simulink model "L7_Project_218"  (R2021b)
settings: Solver=VariableStepAuto  StartTime=0.0  StopTime=0.2  RelTol=1e-3
values from neighbouring files (symbols this model uses):
  Ts = T_pwm    (= 0.001)    [RLagent.m]
  Ts_agent = Ts    (= 0.001)    [RLagent.m]
  Ts_simulink = T_pwm/2    (= 0.0005)    [RLagent.m]
  Ts_speed = 10*Ts    (= 0.01)    [RLagent.m]
undefined symbols (not defined in the file or in its folder): DiscIntNeverNeededParam
libraries: spsIGBTLib x6, spsSeriesRLCBranchLib x6, mcbcontrolslib x3, simulink x2, spsDCVoltageSourceLib x1, spsPermanentMagnetSynchronousMachineLib x1, eePmsmTorqueEstimator x1, rllib x1, spsThreePhaseVIMeasurementLib x1, spspowerguiLib x1
settings Model: Creator=HP  LastModifiedBy=HP
settings DebuggingCC: ParameterPrecisionLossMsg=none

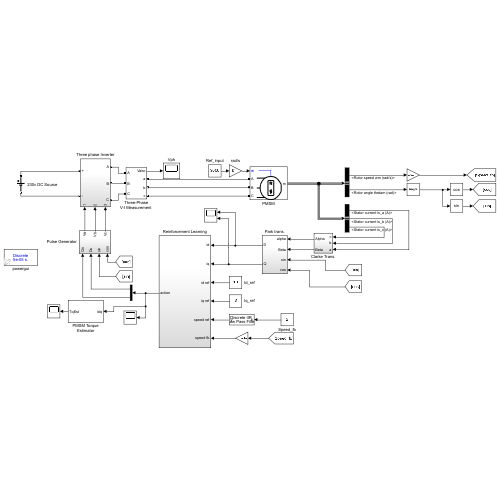
[thumbnail: Simulink's stored preview of the top-level diagram]
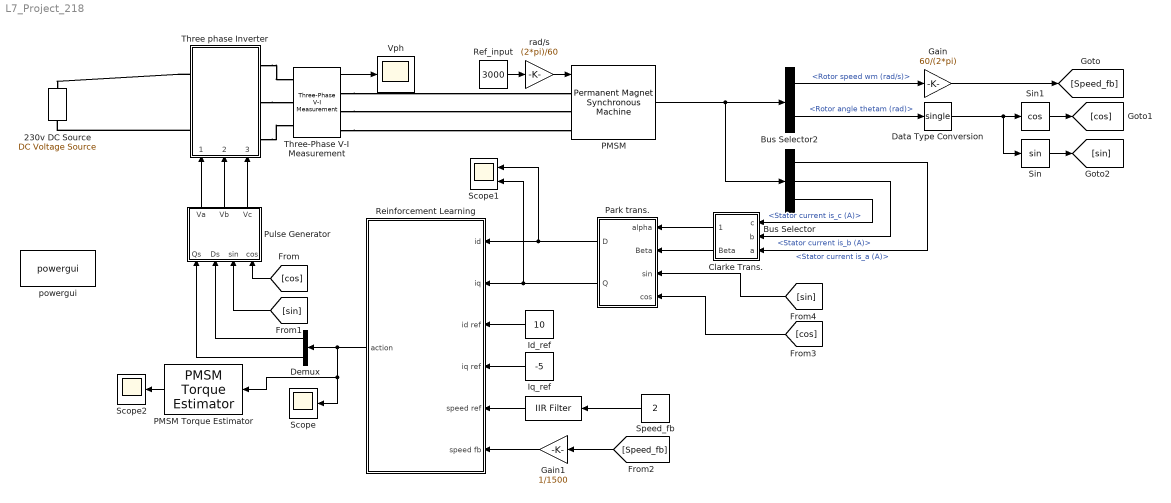
== system L7_Project_218 ==
  "   " : mcbcontrolslib/IIR Filter  VariantControl=Low Pass Filter  VariantSelect=Low-pass  Filter_constant=0.01*(Ts_speed/Ts)  advancedSettings=off  Ts=50e-6  cutOff_freq=353.6777
      settings: SourceProductBaseCode=MT
  230v DC Source : spsDCVoltageSourceLib/DC Voltage Source  Amplitude=230  Measurements=None
  Bus Selector : BusSelector  OutputSignals=Stator current is_a (A),Stator current is_b (A),Stator current is_c (A)
  Bus Selector2 : BusSelector  OutputSignals=Rotor speed wm (rad/s),Rotor angle thetam (rad)
  Clarke Trans. : Subsystem
  Data Type Conversion : DataTypeConversion  OutDataTypeStr=single
  Demux : Demux  Outputs=2
  Gain : Gain  Gain=60/(2*pi)  OutDataTypeStr=double
  Gain1 : Gain  Gain=1/1500
  Id_ref : Constant  Value=10  OutDataTypeStr=double  SampleTime=Ts_speed
  Iq_ref : Constant  Value=-5  OutDataTypeStr=double  SampleTime=Ts_speed
  PMSM : spsPermanentMagnetSynchronousMachineLib/Permanent Magnet Synchronous Machine  NbPhases=3  FluxDistribution=Sinusoidal  RotorType=Salient-pole  MechanicalLoad=Speed w  PresetModel=No  ShowDetailedParameters=on  MeasurementBus=off  Resistance=18.7  Inductance=8.5e-3  dqInductances=[0.02547 0.02816]  La=0.000395  MachineConstant=Flux linkage established by magnets (V.s)  Flux=0.1716  VoltageCst=62.2496  TorqueCst=0.5148  Flat=120  Mechanical=[2.26e-05 1.349e-05 2 0]  PolePairs=2  InitialConditions=[0,0, 0,0]  InitialConditions5ph=[0 0 0 0 0 0]  RefAngle=Aligned with phase A axis (original Park)  IterativeDiscreteModel=Trapezoidal non iterative  TsBlock=-1  TsPowergui=0
  PMSM Torque Estimator : eePmsmTorqueEstimator/PMSM Torque Estimator  ParamType=Constant parameters  p=8  idVect=[-200, 200]  iqVect=[-200, 200]  LdMatrix=0.0002 * ones(2, 2)  LqMatrix=0.0002 * ones(2, 2)  psimMatrix=0.04 * ones(2, 2)  Ld=0.0002  Lq=0.0002  psim=0.04  Ts=-1
      settings: SourceProductBaseCode=PS
  Park trans. : Subsystem
  Pulse Generator : Subsystem
  Ref_input : Constant  Value=3000  SampleTime=Ts_simulink
  Reinforcement Learning : Subsystem
  Scope : Scope
  Scope1 : Scope  NumInputPorts=2
  Scope2 : Scope
  Sin : Trigonometry  NumberOfDataPoints=double
  Sin1 : Trigonometry  Operator=cos
  Speed_fb : Constant  Value=2  SampleTime=Ts_speed
  Three phase Inverter : Subsystem
      settings: PortSchema="{\"entries\":[{\"content\":{\"sides\":[{\"content\":{\"connectorIds\":[\"LConn1\",\"LConn2\"]},\"type\":\"ConnectorPlacement.EquallySpacedRectSide\",\"uuid\":\"7b196236-775e-42c1-83d0-0d6d250710e6\"},{\"content\":{\"connectorIds\":[\"RConn1\",\"RConn2\",\"RConn3\"],\"side\":\"RIGHT\"},\"type\":\"ConnectorPlacement.EquallySpacedRectSide\",\"uuid\":\"b457e177-0c4c-43e7-9cb7-fdd2074136b6\"},{\"content\":{\"connectorIds\":[],\"side\":\"TOP\"},\"type\":\"ConnectorPlacement.EquallySpacedRectSide\",\"uuid\":\"18a8f709-510a-4ef1-9b8b-174ec6aa79c3\"},{\"content\":{\"connectorIds\":[\"In1\",\"In2\",\"In3\"],\"side\":\"BOTTOM\"},\"type\":\"ConnectorPlacement.EquallySpacedRectSide\",\"uuid\":\"6b6fe34a-9a26-41fc-be3f-ad32a70b0e9c\"}]},\"type\":\"ConnectorPlacement.EquallySpacedConnector\",\"uuid\":\"c4aeab25-f1ae-4405-83d3-42d09976eee9\"}],\"packageUris\":[\"http://schema.mathworks.com/mf0/Connector/R2020b\"],\"version\":\"1.0\"}"
  "Three-Phase V-I Measurement " : spsThreePhaseVIMeasurementLib/Three-Phase V-I Measurement  VoltageMeasurement=phase-to-phase  SetLabelV=off  LabelV=Vabc  Vpu=off  VpuLL=off  CurrentMeasurement=no  SetLabelI=off  LabelI=Iabc  Ipu=off  Pbase=100e6  Vbase=500e3  OutputType=Complex  PhasorSimulation=off  PSBequivalent=0
  Vph : Scope
  powergui : spspowerguiLib/powergui  Priority=1  SimulationMode=Discrete  SampleTime=50e-6  frequency=60  Iterations=50  frequencyindice=0  Pbase=100e6  ErrMax=1e-4  UnitsV=kV  UnitsW=MW  buscounter=0  FunctionMessages=off  echomessages=off  EnableUseOfTLC=off  CurrentSourceSwitches=off  DisableSnubberDevices=off  DisableRonSwitches=off  DisableVfSwitches=off  DisplayEquations=off  AutomaticDiscreteSolvers=off  SolverType=Tustin/Backward Euler (TBE)  Interpol=off  ExternalGateDelay=off  methode=off  Ts=100  x0status=blocks  SPID=on  SwTol=0  HookPort=off  NonlinearTolerance=1e-4  nMaxIteration=100  ContinueOnMaxIteration=off  RestoreLinks=warning  ResistiveCurrentMeasurement=off  Frange=[0:2:500]  Ylog=off  Xlog=on  ShowGrid=off  save=off  variable=ZData  structure=0  ZoomFFT=off  StartTime=0.0  cycles=1  DisplayStyle=1  fundamental=60  FreqAxis=off  MaxFrequency=1000  frequencyindicesteady=1  RmsSteady=1  display=off
  rad/s : Gain  Gain=(2*pi)/60  OutDataTypeStr=double
  wires:
  Id_ref/1 -> Reinforcement Learning/3(id ref)
  Clarke Trans./1(Alpha) -> Park trans./1(alpha)
  Speed_fb/1 -> "   "/1
  Bus Selector2/1 -> Gain/1  "<Rotor speed wm (rad/s)>"
  Park trans./2(Q) -> Scope1/2, Reinforcement Learning/2(iq)
  Gain/1 -> [Speed_fb]
  "   "/1 -> Reinforcement Learning/5(speed ref)
  Iq_ref/1 -> Reinforcement Learning/4(iq ref)
  Park trans./1(D) -> Scope1/1, Reinforcement Learning/1(id)
  Clarke Trans./2(Beta) -> Park trans./2(Beta)
  Bus Selector2/2 -> Data Type Conversion/1  "<Rotor angle thetam (rad)>"
  Bus Selector/2 -> Clarke Trans./2(b)  "<Stator current is_b (A)>"
  PMSM/1 -> Bus Selector/1, Bus Selector2/1
  Bus Selector/3 -> Clarke Trans./1(c)  "<Stator current is_c (A)>"
  Bus Selector/1 -> Clarke Trans./3(a)  "<Stator current is_a (A)>"
  Reinforcement Learning/1(action) -> PMSM Torque Estimator/1, Scope/1, Demux/1
  Demux/1 -> Pulse Generator/2(Ds)
  Demux/2 -> Pulse Generator/1(Qs)
  Pulse Generator/1(Va) -> Three phase Inverter/1(1)
  Pulse Generator/2(Vb) -> Three phase Inverter/2(2)
  Pulse Generator/3(Vc) -> Three phase Inverter/3(3)
  Data Type Conversion/1 -> Sin/1, Sin1/1
  Sin1/1 -> [cos]
  Sin/1 -> [sin]
  [cos] -> Pulse Generator/4(cos)
  [sin] -> Pulse Generator/3(sin)
  [Speed_fb] -> Gain1/1
  [cos] -> Park trans./4(cos)
  [sin] -> Park trans./3(sin)
  "Three-Phase V-I Measurement "/1 -> Vph/1
  Gain1/1 -> Reinforcement Learning/6(speed fb)
  Ref_input/1 -> rad/s/1
  PMSM Torque Estimator/1 -> Scope2/1
  rad/s/1 -> PMSM/1
  connections:
  Three phase Inverter/LConn2 -- 230v DC Source/LConn1
  Three phase Inverter/LConn1 -- 230v DC Source/RConn1
  Three phase Inverter/RConn2 -- "Three-Phase V-I Measurement "/LConn2
  Three phase Inverter/RConn1 -- "Three-Phase V-I Measurement "/LConn1
  Three phase Inverter/RConn3 -- "Three-Phase V-I Measurement "/LConn3
  "Three-Phase V-I Measurement "/RConn1 -- PMSM/LConn1
  "Three-Phase V-I Measurement "/RConn2 -- PMSM/LConn2
  "Three-Phase V-I Measurement "/RConn3 -- PMSM/LConn3

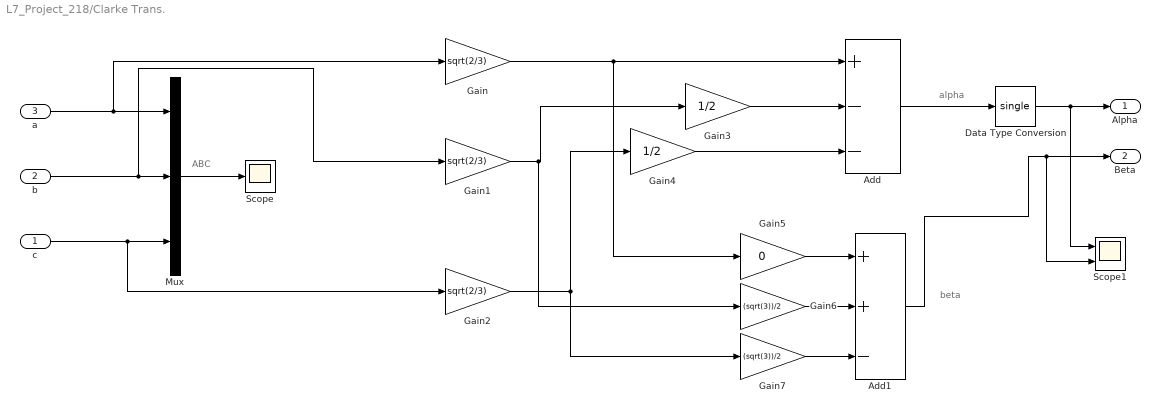
== system L7_Project_218/Clarke Trans. ==
  note: ABC
  note: beta
  note: alpha
  c : Inport
  b : Inport  Port=2
  a : Inport  Port=3
  Add : Sum  Inputs=+--  AccumDataTypeStr=single
  Add1 : Sum  Inputs=++-  AccumDataTypeStr=double
  Data Type Conversion : DataTypeConversion  OutDataTypeStr=single
  Gain : Gain  Gain=sqrt(2/3)
  Gain1 : Gain  Gain=sqrt(2/3)
  Gain2 : Gain  Gain=sqrt(2/3)
  Gain3 : Gain  Gain=1/2
  Gain4 : Gain  Gain=1/2
  Gain5 : Gain  Gain=0
  Gain6 : Gain  Gain=(sqrt(3))/2
  Gain7 : Gain  Gain=(sqrt(3))/2
  Mux : Mux  Inputs=3
  Scope : Scope
  Scope1 : Scope  NumInputPorts=2
  Alpha : Outport
  Beta : Outport  Port=2
  wires:
  Gain2/1 -> Gain4/1, Gain7/1
  Gain/1 -> Gain5/1, Add/1
  Gain1/1 -> Gain6/1, Gain3/1
  Gain6/1 -> Add1/2
  a/1 -> Gain/1, Mux/1
  b/1 -> Gain1/1, Mux/2
  c/1 -> Gain2/1, Mux/3
  Gain5/1 -> Add1/1
  Gain7/1 -> Add1/3
  Gain3/1 -> Add/2
  Gain4/1 -> Add/3
  Mux/1 -> Scope/1
  Add1/1 -> Scope1/2, Beta/1
  Add/1 -> Data Type Conversion/1
  Data Type Conversion/1 -> Scope1/1, Alpha/1

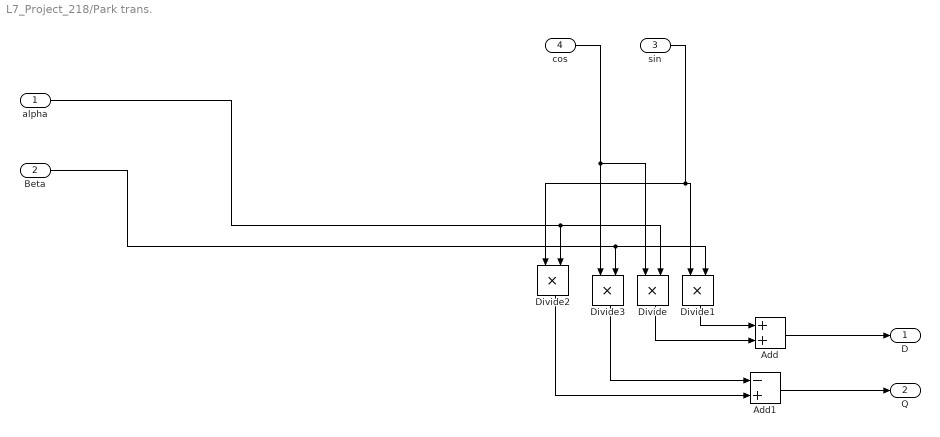
== system L7_Project_218/Park trans. ==
  alpha : Inport
  Beta : Inport  Port=2
  sin : Inport  Port=3
  cos : Inport  Port=4
  Add : Sum
  Add1 : Sum  Inputs=-+
  Divide{,1..3} (4 alike) : Product  Inputs=**
  D : Outport
  Q : Outport  Port=2
  wires:
  cos/1 -> Divide/1, Divide3/1
  Divide3/1 -> Add1/1
  alpha/1 -> Divide2/2, Divide/2
  Divide1/1 -> Add/1
  sin/1 -> Divide2/1, Divide1/1
  Add1/1 -> Q/1
  Divide/1 -> Add/2
  Divide2/1 -> Add1/2
  Beta/1 -> Divide3/2, Divide1/2
  Add/1 -> D/1

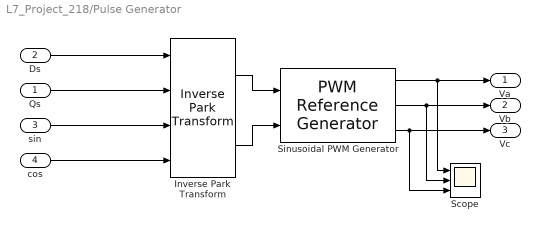
== system L7_Project_218/Pulse Generator ==
  Qs : Inport
  Ds : Inport  Port=2
  sin : Inport  Port=3
  cos : Inport  Port=4
  Inverse Park Transform : mcbcontrolslib/Inverse Park Transform  AxisAlignment=D-axis
  Scope : Scope  NumInputPorts=3
  Sinusoidal PWM Generator : mcbcontrolslib/PWM Reference Generator  inSignal=Valphabeta  modType=SPWM: sinusoidal PWM
      settings: SourceProductBaseCode=MT
  Va : Outport
  Vb : Outport  Port=2
  Vc : Outport  Port=3
  wires:
  Inverse Park Transform/2 -> Sinusoidal PWM Generator/2
  Inverse Park Transform/1 -> Sinusoidal PWM Generator/1
  cos/1 -> Inverse Park Transform/4
  Qs/1 -> Inverse Park Transform/2
  sin/1 -> Inverse Park Transform/3
  Ds/1 -> Inverse Park Transform/1
  Sinusoidal PWM Generator/1 -> Scope/1, Va/1
  Sinusoidal PWM Generator/2 -> Scope/2, Vb/1
  Sinusoidal PWM Generator/3 -> Scope/3, Vc/1

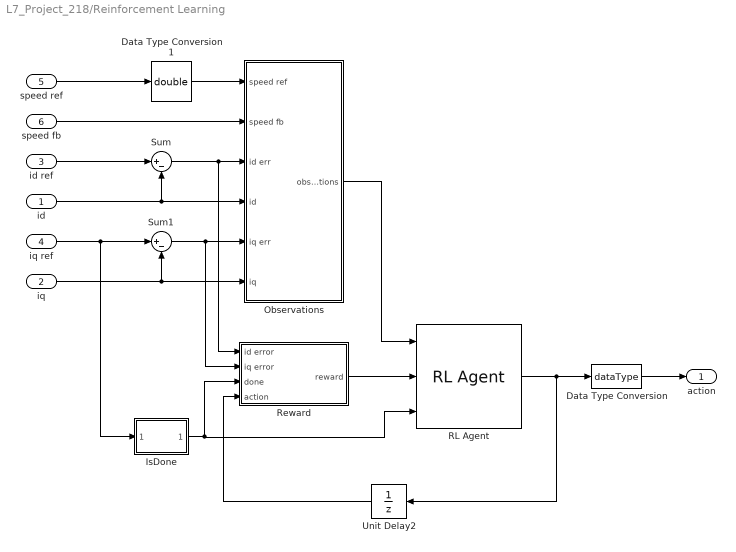
== system L7_Project_218/Reinforcement Learning ==
  id : Inport
  iq : Inport  Port=2
  id ref : Inport  Port=3
  iq ref : Inport  Port=4
  speed ref : Inport  Port=5
  speed fb : Inport  Port=6
  Data Type Conversion : DataTypeConversion  OutDataTypeStr=dataType
  Data Type Conversion1 : DataTypeConversion  OutDataTypeStr=double
  IsDone : Subsystem
  Observations : Subsystem
  RL Agent : rllib/RL Agent  Agent=agent  ExternalActionAsInput=off  ProvideCumRwd=off  TreatAsDirectFeedthrough=on
  Reward : Subsystem
  Sum : Sum  Inputs=|+-  OutDataTypeStr=Inherit: Inherit via back propagation
  Sum1 : Sum  Inputs=|+-  OutDataTypeStr=Inherit: Inherit via back propagation
  Unit Delay2 : UnitDelay  SampleTime=-1  HasFrameUpgradeWarning=on
  action : Outport
  wires:
  Sum1/1 -> Reward/2(iq error), Observations/5(iq err)
  Sum/1 -> Reward/1(id error), Observations/3(id err)
  iq/1 -> Sum1/2, Observations/6(iq)
  speed fb/1 -> Observations/2(speed fb)
  speed ref/1 -> Data Type Conversion1/1
  Reward/1(reward) -> RL Agent/2
  Observations/1(observations) -> RL Agent/1
  iq ref/1 -> IsDone/1(Iq_ref), Sum1/1
  id/1 -> Sum/2, Observations/4(id)
  id ref/1 -> Sum/1
  Unit Delay2/1 -> Reward/4(action)
  RL Agent/1 -> Data Type Conversion/1, Unit Delay2/1
  IsDone/1(stop) -> RL Agent/3, Reward/3(done)
  Data Type Conversion/1 -> action/1
  Data Type Conversion1/1 -> Observations/1(speed ref)

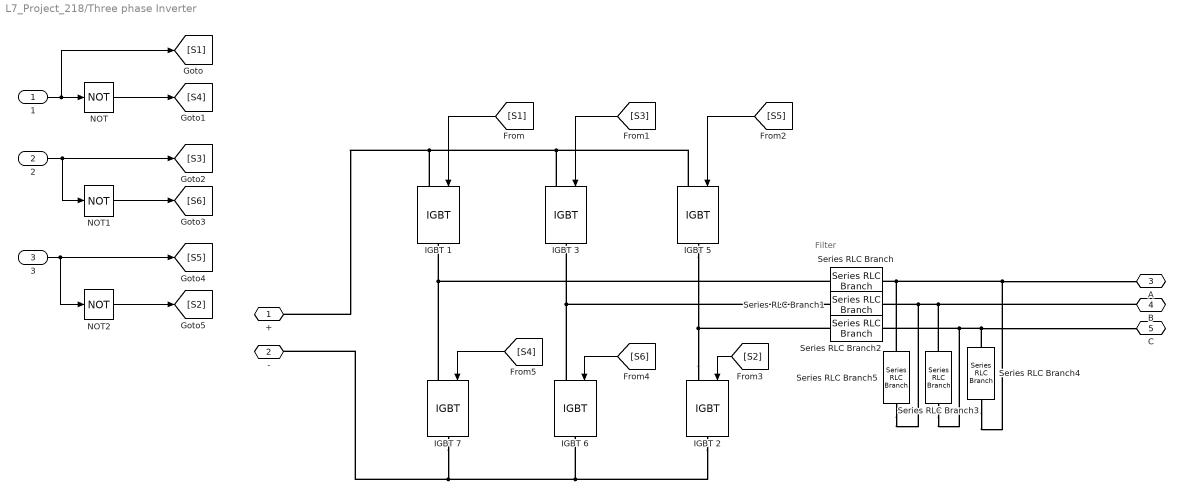
== system L7_Project_218/Three phase Inverter ==
  note: Filter
  1 : Inport
  2 : Inport  Port=2
  3 : Inport  Port=3
  IGBT {1..3,5..7} (6 alike) : spsIGBTLib/IGBT  Ron=0.001  Lon=0  Vf=1  Tf=1e-6  Tt=2e-6  IC=0  Rs=1e5  Cs=inf  Measurements=off
  NOT : Logic  Operator=NOT  IconShape=distinctive  AllPortsSameDT=off  OutDataTypeStr=boolean
  NOT1 : Logic  Operator=NOT  IconShape=distinctive  AllPortsSameDT=off  OutDataTypeStr=boolean
  NOT2 : Logic  Operator=NOT  IconShape=distinctive  AllPortsSameDT=off  OutDataTypeStr=boolean
  Series RLC Branch : spsSeriesRLCBranchLib/Series RLC Branch  LConnTagsString=__new0  RConnTagsString=__new0  BranchType=L  Resistance=1  Inductance=470e-6  SetiL0=off  InitialCurrent=0  Capacitance=1e-6  Setx0=off  InitialVoltage=0  Measurements=None
  Series RLC Branch1 : spsSeriesRLCBranchLib/Series RLC Branch  LConnTagsString=__new0  RConnTagsString=__new0  BranchType=L  Resistance=1  Inductance=470e-6  SetiL0=off  InitialCurrent=0  Capacitance=1e-6  Setx0=off  InitialVoltage=0  Measurements=None
  Series RLC Branch2 : spsSeriesRLCBranchLib/Series RLC Branch  LConnTagsString=__new0  RConnTagsString=__new0  BranchType=L  Resistance=1  Inductance=470e-6  SetiL0=off  InitialCurrent=0  Capacitance=1e-6  Setx0=off  InitialVoltage=0  Measurements=None
  Series RLC Branch3 : spsSeriesRLCBranchLib/Series RLC Branch  LConnTagsString=__new0  RConnTagsString=__new0  BranchType=C  Resistance=1  Inductance=1e-3  SetiL0=off  InitialCurrent=0  Capacitance=1e-6  Setx0=off  InitialVoltage=0  Measurements=None
  Series RLC Branch4 : spsSeriesRLCBranchLib/Series RLC Branch  LConnTagsString=__new0  RConnTagsString=__new0  BranchType=C  Resistance=1  Inductance=1e-3  SetiL0=off  InitialCurrent=0  Capacitance=1e-6  Setx0=off  InitialVoltage=0  Measurements=None
  Series RLC Branch5 : spsSeriesRLCBranchLib/Series RLC Branch  LConnTagsString=__new0  RConnTagsString=__new0  BranchType=C  Resistance=1  Inductance=1e-3  SetiL0=off  InitialCurrent=0  Capacitance=1e-6  Setx0=off  InitialVoltage=0  Measurements=None
  + : PMIOPort  Side=Left
  - : PMIOPort  Port=2  Side=Left
  A : PMIOPort  Port=3  Side=Right
  B : PMIOPort  Port=4  Side=Right
  C : PMIOPort  Port=5  Side=Right
  wires:
  [S3] -> IGBT 3/1
  [S1] -> IGBT 1/1
  [S5] -> IGBT 5/1
  [S4] -> IGBT 7/1
  [S6] -> IGBT 6/1
  [S2] -> IGBT 2/1
  1/1 -> [S1], NOT/1
  NOT/1 -> [S4]
  2/1 -> [S3], NOT1/1
  NOT1/1 -> [S6]
  3/1 -> NOT2/1, [S5]
  NOT2/1 -> [S2]
  connections:
  IGBT 3/RConn1 -- Series RLC Branch1/LConn1 -- IGBT 6/LConn1
  IGBT 6/RConn1 -- IGBT 2/RConn1 -- IGBT 7/RConn1 -- -/RConn1
  Series RLC Branch2/RConn1 -- Series RLC Branch3/RConn1 -- Series RLC Branch4/LConn1 -- C/RConn1
  IGBT 1/RConn1 -- Series RLC Branch/LConn1 -- IGBT 7/LConn1
  IGBT 5/LConn1 -- IGBT 3/LConn1 -- IGBT 1/LConn1 -- +/RConn1
  IGBT 2/LConn1 -- Series RLC Branch2/LConn1 -- IGBT 5/RConn1
  Series RLC Branch4/RConn1 -- A/RConn1 -- Series RLC Branch/RConn1 -- Series RLC Branch5/LConn1
  Series RLC Branch1/RConn1 -- Series RLC Branch5/RConn1 -- B/RConn1 -- Series RLC Branch3/LConn1

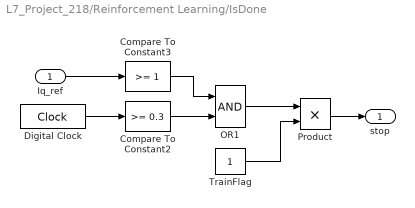
== system L7_Project_218/Reinforcement Learning/IsDone ==
  Iq_ref : Inport
  Compare To Constant2 : simulink/Logic and Bit Operations/Compare To Constant  relop=>=  const=0.3  OutDataTypeStr=boolean
  Compare To Constant3 : simulink/Logic and Bit Operations/Compare To Constant  relop=>=  const=1  OutDataTypeStr=boolean
  Digital Clock : DigitalClock  SampleTime=Ts_agent
  OR1 : Logic  IconShape=distinctive  AllPortsSameDT=off  OutDataTypeStr=boolean
  Product : Product
  TrainFlag : Constant  OutDataTypeStr=double
  stop : Outport
  wires:
  Compare To Constant2/1 -> OR1/2
  Iq_ref/1 -> Compare To Constant3/1
  Compare To Constant3/1 -> OR1/1
  OR1/1 -> Product/1
  Digital Clock/1 -> Compare To Constant2/1
  Product/1 -> stop/1
  TrainFlag/1 -> Product/2

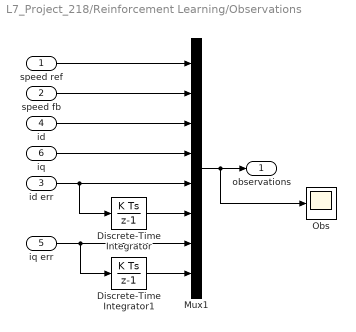
== system L7_Project_218/Reinforcement Learning/Observations ==
  speed ref : Inport
  speed fb : Inport  Port=2
  id err : Inport  Port=3
  id : Inport  Port=4
  iq err : Inport  Port=5
  iq : Inport  Port=6
  Discrete-Time Integrator : DiscreteIntegrator  SampleTime=-1  ICPrevOutput=DiscIntNeverNeededParam  ICPrevScaledInput=DiscIntNeverNeededParam
  Discrete-Time Integrator1 : DiscreteIntegrator  SampleTime=-1  ICPrevOutput=DiscIntNeverNeededParam  ICPrevScaledInput=DiscIntNeverNeededParam
  Mux1 : Mux  Inputs=8
  Obs : Scope
  observations : Outport  VectorParamsAs1DForOutWhenUnconnected=off
  wires:
  speed ref/1 -> Mux1/1
  speed fb/1 -> Mux1/2
  id/1 -> Mux1/3
  iq/1 -> Mux1/4
  Mux1/1 -> Obs/1, observations/1
  Discrete-Time Integrator1/1 -> Mux1/8
  iq err/1 -> Mux1/7, Discrete-Time Integrator1/1
  Discrete-Time Integrator/1 -> Mux1/6
  id err/1 -> Mux1/5, Discrete-Time Integrator/1

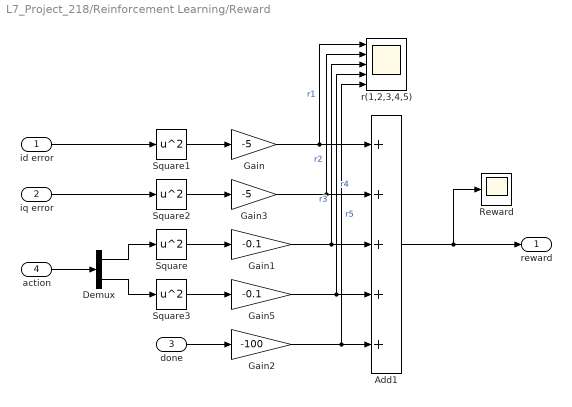
== system L7_Project_218/Reinforcement Learning/Reward ==
  id error : Inport
  iq error : Inport  Port=2
  done : Inport  Port=3
  action : Inport  Port=4
  " r(1,2,3,4,5)" : Scope  NumInputPorts=5
  Add1 : Sum  Inputs=+++++
  Demux : Demux  Outputs=2
  Gain : Gain  Gain=-5
  Gain1 : Gain  Gain=-0.1
  Gain2 : Gain  Gain=-100
  Gain3 : Gain  Gain=-5
  Gain5 : Gain  Gain=-0.1
  Reward : Scope
  Square{,1..3} (4 alike) : Math  Operator=square  SaturateOnIntegerOverflow=on
  reward : Outport  VectorParamsAs1DForOutWhenUnconnected=off
  wires:
  Square1/1 -> Gain/1
  Square2/1 -> Gain3/1
  Demux/1 -> Square/1
  Square/1 -> Gain1/1
  Gain1/1 -> " r(1,2,3,4,5)"/3, Add1/3  "r3"
  Demux/2 -> Square3/1
  Square3/1 -> Gain5/1
  action/1 -> Demux/1
  Add1/1 -> Reward/1, reward/1
  Gain5/1 -> " r(1,2,3,4,5)"/4, Add1/4  "r4"
  Gain/1 -> " r(1,2,3,4,5)"/1, Add1/1  "r1"
  Gain3/1 -> " r(1,2,3,4,5)"/2, Add1/2  "r2"
  id error/1 -> Square1/1
  iq error/1 -> Square2/1
  Gain2/1 -> Add1/5, " r(1,2,3,4,5)"/5  "r5"
  done/1 -> Gain2/1
